simulink model "Lab1_3_eje2_comp_CdyCz"  (R2023b)
settings: Solver=VariableStepAuto  StartTime=0.0  StopTime=2.0  RelTol=1e-3
undefined symbols (not defined in the file or in its folder): a1z, a2z, b0z, b1z, b2z, d1, d2, p, q, qd1, r, rd1d2, Ts
libraries: cstblocks x5
settings Model: Creator=chris  LastModifiedBy=chris

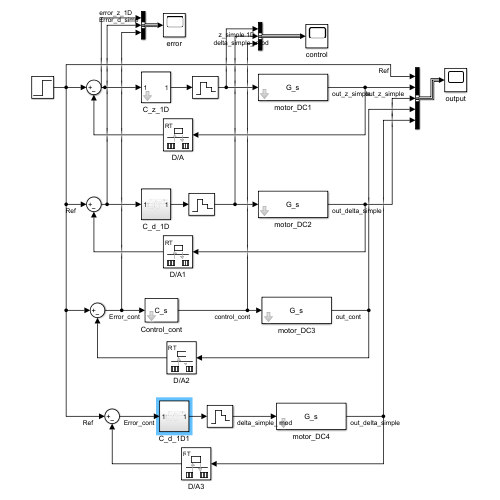
[thumbnail: Simulink's stored preview of the top-level diagram]
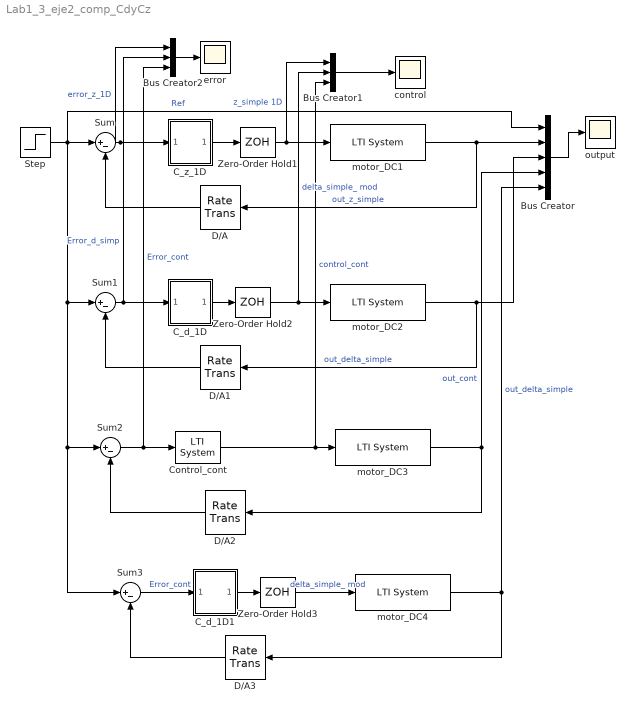
== system Lab1_3_eje2_comp_CdyCz ==
  Bus Creator : BusCreator  Inputs=5
  Bus Creator1 : BusCreator  Inputs=3
  Bus Creator2 : BusCreator  Inputs=3
  C_d_1D : Subsystem
  C_d_1D1 : Subsystem
  C_z_1D : Subsystem  mask{b0z=b0z, b1z=b1z, b2z=b2z, a1z=a1z, a2z=a2z}
  Control_cont : cstblocks/LTI System  sys=C_s  IC=[]  PadeOrder=0
  D/A{,1..3} (4 alike) : RateTransition  Priority=0  Integrity=off  Deterministic=off  OutPortSampleTime=Ts
  Step : Step  Time=0.2  SampleTime=0
  Sum{,1..3} (4 alike) : Sum  Inputs=|+-
  Zero-Order Hold1 : ZeroOrderHold  SampleTime=-1
  Zero-Order Hold2 : ZeroOrderHold  SampleTime=Ts
  Zero-Order Hold3 : ZeroOrderHold  SampleTime=Ts
  control : Scope
  error : Scope
  motor_DC{1..4} (4 alike) : cstblocks/LTI System  sys=G_s  IC=[]  PadeOrder=0
  output : Scope
  wires:
  Sum/1 -> C_z_1D/1(In1), Bus Creator2/1  "error_z_1D"
  C_z_1D/1(Out1) -> Zero-Order Hold1/1
  motor_DC1/1 -> D/A/1, Bus Creator/2  "out_z_simple"
  D/A/1 -> Sum/2
  Bus Creator/1 -> output/1
  motor_DC2/1 -> Bus Creator/3, D/A1/1  "out_delta_simple"
  D/A1/1 -> Sum1/2
  Zero-Order Hold2/1 -> Bus Creator1/2, motor_DC2/1  "delta_simple_ mod"
  C_d_1D/1(Out1) -> Zero-Order Hold2/1
  Sum1/1 -> C_d_1D/1(In1), Bus Creator2/2  "Error_d_simp"
  Bus Creator1/1 -> control/1
  Bus Creator2/1 -> error/1
  Zero-Order Hold1/1 -> Bus Creator1/1, motor_DC1/1  "z_simple 1D"
  Sum2/1 -> Bus Creator2/3, Control_cont/1  "Error_cont"
  D/A2/1 -> Sum2/2
  motor_DC3/1 -> Bus Creator/4, D/A2/1  "out_cont"
  Control_cont/1 -> Bus Creator1/3, motor_DC3/1  "control_cont"
  Step/1 -> Sum3/1, Sum2/1, Sum1/1, Bus Creator/1, Sum/1  "Ref"
  Sum3/1 -> C_d_1D1/1(In1)  "Error_cont"
  D/A3/1 -> Sum3/2
  Zero-Order Hold3/1 -> motor_DC4/1  "delta_simple_ mod"
  motor_DC4/1 -> Bus Creator/5, D/A3/1  "out_delta_simple"
  C_d_1D1/1(Out1) -> Zero-Order Hold3/1

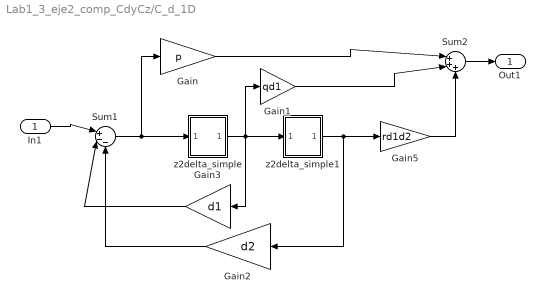
== system Lab1_3_eje2_comp_CdyCz/C_d_1D ==
  In1 : Inport
  Gain : Gain  Gain=p
  Gain1 : Gain  Gain=qd1
  Gain2 : Gain  Gain=d2
  Gain3 : Gain  Gain=d1
  Gain5 : Gain  Gain=rd1d2
  Sum1 : Sum  Inputs=|+--
  Sum2 : Sum  Inputs=|+++
  z2delta_simple : Subsystem
  z2delta_simple1 : Subsystem
  Out1 : Outport
  wires:
  In1/1 -> Sum1/1
  Gain1/1 -> Sum2/2
  Gain5/1 -> Sum2/3
  Gain/1 -> Sum2/1
  Sum2/1 -> Out1/1
  z2delta_simple1/1(Out1) -> Gain2/1, Gain5/1
  Sum1/1 -> z2delta_simple/1(In1), Gain/1
  z2delta_simple/1(Out1) -> Gain3/1, z2delta_simple1/1(In1), Gain1/1
  Gain3/1 -> Sum1/2
  Gain2/1 -> Sum1/3

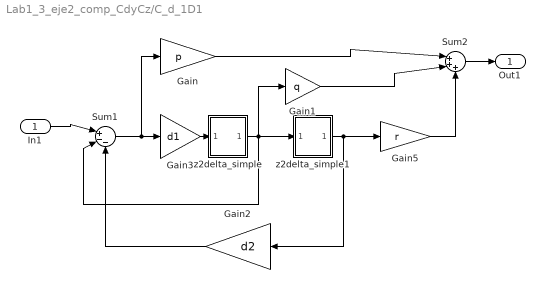
== system Lab1_3_eje2_comp_CdyCz/C_d_1D1 ==
  In1 : Inport
  Gain : Gain  Gain=p
  Gain1 : Gain  Gain=q
  Gain2 : Gain  Gain=d2
  Gain3 : Gain  Gain=d1
  Gain5 : Gain  Gain=r
  Sum1 : Sum  Inputs=|+--
  Sum2 : Sum  Inputs=|+++
  z2delta_simple : Subsystem
  z2delta_simple1 : Subsystem
  Out1 : Outport
  wires:
  In1/1 -> Sum1/1
  Gain1/1 -> Sum2/2
  Gain5/1 -> Sum2/3
  Gain/1 -> Sum2/1
  Sum2/1 -> Out1/1
  z2delta_simple1/1(Out1) -> Gain2/1, Gain5/1
  Sum1/1 -> Gain/1, Gain3/1
  z2delta_simple/1(Out1) -> Gain1/1, Sum1/2, z2delta_simple1/1(In1)
  Gain2/1 -> Sum1/3
  Gain3/1 -> z2delta_simple/1(In1)

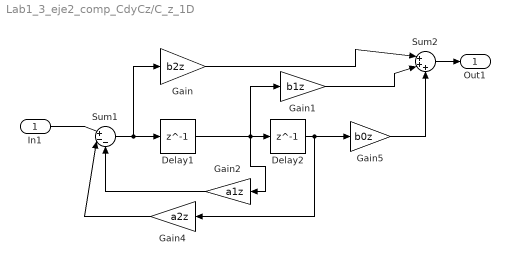
== system Lab1_3_eje2_comp_CdyCz/C_z_1D ==
  In1 : Inport
  Delay1 : Delay  DelayLength=1  InitialCondition=0
  Delay2 : Delay  DelayLength=1  InitialCondition=0
  Gain : Gain  Gain=b2z
  Gain1 : Gain  Gain=b1z
  Gain2 : Gain  Gain=a1z
  Gain4 : Gain  Gain=a2z
  Gain5 : Gain  Gain=b0z
  Sum1 : Sum  Inputs=|+--
  Sum2 : Sum  Inputs=|+++
  Out1 : Outport
  wires:
  Delay2/1 -> Gain5/1, Gain4/1
  Gain4/1 -> Sum1/2
  Delay1/1 -> Gain1/1, Gain2/1, Delay2/1
  In1/1 -> Sum1/1
  Gain1/1 -> Sum2/2
  Gain5/1 -> Sum2/3
  Gain/1 -> Sum2/1
  Sum2/1 -> Out1/1
  Gain2/1 -> Sum1/3
  Sum1/1 -> Gain/1, Delay1/1

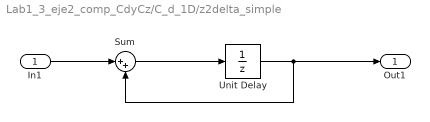
== system Lab1_3_eje2_comp_CdyCz/C_d_1D/z2delta_simple ==
  In1 : Inport
  Sum : Sum  Inputs=|++
  Unit Delay : UnitDelay  SampleTime=-1  HasFrameUpgradeWarning=on
  Out1 : Outport
  wires:
  In1/1 -> Sum/1
  Unit Delay/1 -> Out1/1, Sum/2
  Sum/1 -> Unit Delay/1

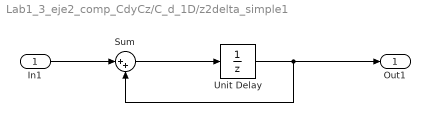
== system Lab1_3_eje2_comp_CdyCz/C_d_1D/z2delta_simple1 ==
  In1 : Inport
  Sum : Sum  Inputs=|++
  Unit Delay : UnitDelay  SampleTime=-1  HasFrameUpgradeWarning=on
  Out1 : Outport
  wires:
  In1/1 -> Sum/1
  Unit Delay/1 -> Out1/1, Sum/2
  Sum/1 -> Unit Delay/1

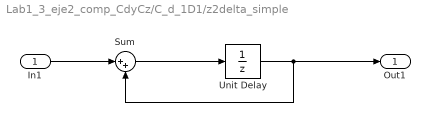
== system Lab1_3_eje2_comp_CdyCz/C_d_1D1/z2delta_simple ==
  In1 : Inport
  Sum : Sum  Inputs=|++
  Unit Delay : UnitDelay  SampleTime=-1  HasFrameUpgradeWarning=on
  Out1 : Outport
  wires:
  In1/1 -> Sum/1
  Unit Delay/1 -> Out1/1, Sum/2
  Sum/1 -> Unit Delay/1

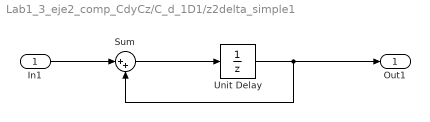
== system Lab1_3_eje2_comp_CdyCz/C_d_1D1/z2delta_simple1 ==
  In1 : Inport
  Sum : Sum  Inputs=|++
  Unit Delay : UnitDelay  SampleTime=-1  HasFrameUpgradeWarning=on
  Out1 : Outport
  wires:
  In1/1 -> Sum/1
  Unit Delay/1 -> Out1/1, Sum/2
  Sum/1 -> Unit Delay/1
